simulink model "toilettenspuelung"  (R2014b)
settings: Solver=ode45  StartTime=0.0  StopTime=10.0  RelTol=1e-3
settings Model: Creator=sigurd  LastModifiedBy=sigurd

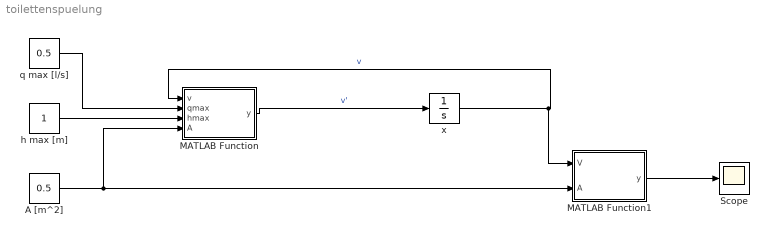
== system toilettenspuelung ==
  A [m^2] : Constant  Value=0.5
  MATLAB Function : MATLAB Function  TreatAsAtomicUnit=on
  MATLAB Function1 : MATLAB Function  TreatAsAtomicUnit=on
  Scope : Scope
  h max [m] : Constant
  q max [l/s] : Constant  Value=0.5
  x : Integrator
  wires:
  MATLAB Function/1(y) -> x/1  "v'"
  x/1 -> MATLAB Function1/1(V), MATLAB Function/1(v)  "v"
  h max [m]/1 -> MATLAB Function/3(hmax)
  q max [l/s]/1 -> MATLAB Function/2(qmax)
  A [m^2]/1 -> MATLAB Function/4(A), MATLAB Function1/2(A)
  MATLAB Function1/1(y) -> Scope/1

== matlab function toilettenspuelung/MATLAB Function1 ==
  data: V input; y output; A input
function y = fcn(V,A)
%#codegen

y = V/A;

== matlab function toilettenspuelung/MATLAB Function ==
  data: v input; y output; qmax input; hmax input; A input
function y = fcn(v,qmax,hmax,A)

y = qmax - (v*(qmax/(hmax*A)));
